simulink model "trajectorygenerator"  (R2016a)
settings: Solver=VariableStepAuto  StartTime=0.0  StopTime=10.0  RelTol=1e-3
settings Model: Creator=hqm3yy  LastModifiedBy=hqm3yy

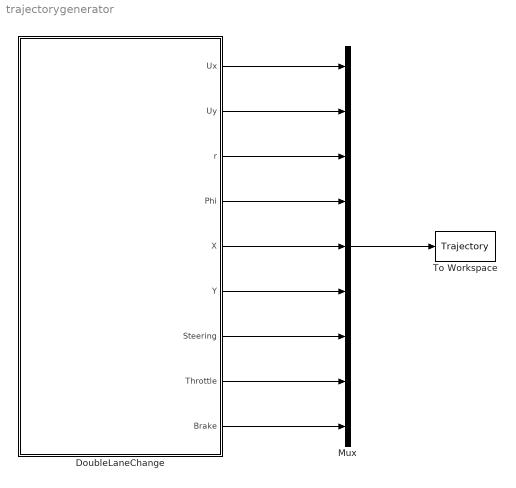
== system trajectorygenerator ==
  DoubleLaneChange : Subsystem  Tag=AME2SLCoSim  InitFcn=AMESimLib_initBlock  StartFcn=AMESimLib_startBlock  StopFcn=AMESimLib_stopBlock
      settings: DeleteFcn=AMESimLib_deleteBlock  OpenFcn=AMESimLib_openBlock('AME2SLCoSim')
      mask Display: image(imread('amesim_pix256.png'),[0.4,0.7,0.2,0.2]);disp('Simcenter Amesim co-Sim:\nDoubleLaneChange');port_label('output',1,'Ux');port_label('output',2,'Uy');port_label('output',3,'r');port_label('output',4,'Phi');port_label('output',5,'X');port_label('output',6,'Y');port_label('output',7,'Steering');port_label('output',8,'Throttle');port_label('output',9,'Brake');
  Mux : Mux  Inputs=9
  To Workspace : ToWorkspace  VariableName=Trajectory  SaveFormat=Timeseries  SampleTime=-1
  wires:
  DoubleLaneChange/1(Ux) -> Mux/1
  DoubleLaneChange/2(Uy) -> Mux/2
  DoubleLaneChange/3(r) -> Mux/3
  DoubleLaneChange/4(Phi) -> Mux/4
  DoubleLaneChange/5(X) -> Mux/5
  DoubleLaneChange/6(Y) -> Mux/6
  DoubleLaneChange/9(Brake) -> Mux/9
  DoubleLaneChange/8(Throttle) -> Mux/8
  DoubleLaneChange/7(Steering) -> Mux/7
  Mux/1 -> To Workspace/1

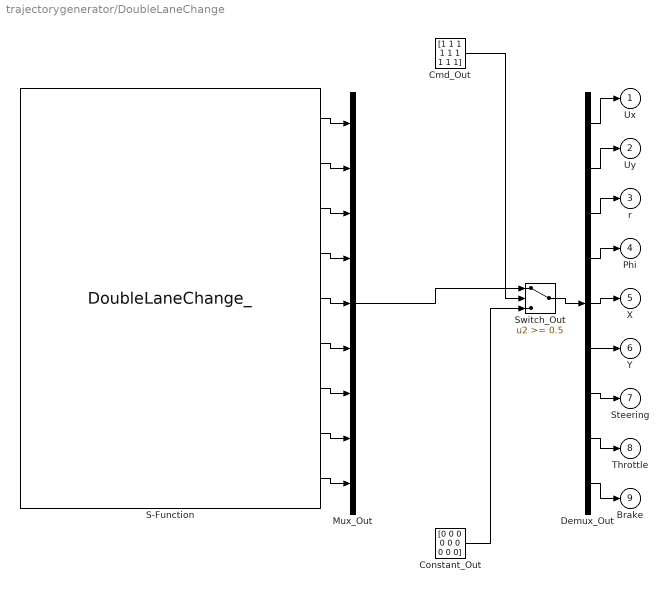
== system trajectorygenerator/DoubleLaneChange ==
  Cmd_Out : Constant  Value=[1 1 1 1 1 1 1 1 1]
  Constant_Out : Constant  Value=[0 0 0 0 0 0 0 0 0]
  Demux_Out : Demux  Outputs=9
  Mux_Out : Mux  Inputs=9
  S-Function : S-Function  InitFcn=clear DoubleLaneChange_  StopFcn=clear DoubleLaneChange_  FunctionName=DoubleLaneChange_  Parameters="[0.01;0.05;1e-05;1e+30;100;0;0;0;0;1;0.001;0;1] ['Grav           ';'Xg             ';'Zg             ';'Msprung        ';'Msteer         ';'Msp_front      ';'Mwh_front      ';'Msp_rear       ';'Mwh_rear       ';'Isprung_xx     ';'Isprung_yy     ';'Isprung_zz     ';'Isprung_xy     ';'Isprung_xz     ';'Isprung_yz     ';'Zref_front     ';'Zref_rear      ';'wheelbase      ';'track_front    ';'track_rear     ';'Rpinion        ';'Ksusp_front    ';'Ksusp_rear     ';'Rsusp_front    ';'Rsusp_rear     ';'Kantiroll_front';'Kantiroll_rear ';'Rfree          ';'Rroll          ';'Ktire          ';'Rtire          ';'a1             ';'a2             ';'a3             ';'a4             '] [9.8066;1056;375;1300;2;18;18;15;14;250;1000;1300;0;-20;0;75;75;2400;1450;1450;8;21000;21000;2000;1500;30000;20000;0.292;0.291;200000;100;-50;1200;1000;5] [] [] [] []"  SFunctionDeploymentMode=off  EnableBusSupport=off
      mask Display: port_label('output',1,'Ux');port_label('output',2,'Uy');port_label('output',3,'r');port_label('output',4,'Phi');port_label('output',5,'X');port_label('output',6,'Y');port_label('output',7,'Steering');port_label('output',8,'Throttle');port_label('output',9,'Brake');disp('Simcenter Amesim:\n DoubleLaneChange_')
  Switch_Out : Switch  Threshold=0.5  SaturateOnIntegerOverflow=on  InputSameDT=on
  Ux : Outport
  Uy : Outport  Port=2
  r : Outport  Port=3
  Phi : Outport  Port=4
  X : Outport  Port=5
  Y : Outport  Port=6
  Steering : Outport  Port=7
  Throttle : Outport  Port=8
  Brake : Outport  Port=9
  wires:
  Mux_Out/1 -> Switch_Out/1
  Cmd_Out/1 -> Switch_Out/2
  Constant_Out/1 -> Switch_Out/3
  Switch_Out/1 -> Demux_Out/1
  Demux_Out/1 -> Ux/1
  S-Function/1 -> Mux_Out/1
  Demux_Out/2 -> Uy/1
  S-Function/2 -> Mux_Out/2
  Demux_Out/3 -> r/1
  S-Function/3 -> Mux_Out/3
  Demux_Out/4 -> Phi/1
  S-Function/4 -> Mux_Out/4
  Demux_Out/5 -> X/1
  S-Function/5 -> Mux_Out/5
  Demux_Out/6 -> Y/1
  S-Function/6 -> Mux_Out/6
  Demux_Out/7 -> Steering/1
  S-Function/7 -> Mux_Out/7
  Demux_Out/8 -> Throttle/1
  S-Function/8 -> Mux_Out/8
  Demux_Out/9 -> Brake/1
  S-Function/9 -> Mux_Out/9
